simulink model "simple_block"  (Simulink 6.0)
settings: Solver=ode3  StartTime=0.0  StopTime=10.0  FixedStep=0.01  RelTol=1e-3
settings Model: LastModifiedBy=Administrator

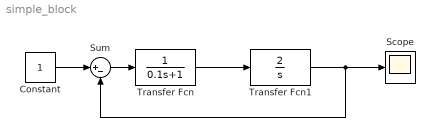
== system simple_block ==
  Constant : Constant
  Scope : Scope
      settings: SaveName=mout  DataFormat=Array
  Sum : Sum  Inputs=|+-
  Transfer Fcn : TransferFcn  Denominator=[0.1 1]
  Transfer Fcn1 : TransferFcn  Numerator=[2]  Denominator=[1 0]
  wires:
  Constant/1 -> Sum/1
  Sum/1 -> Transfer Fcn/1
  Transfer Fcn/1 -> Transfer Fcn1/1
  Transfer Fcn1/1 -> Scope/1, Sum/2
